simulink model "feedBackCtlPractice1"  (R2020b)
settings: Solver=ode4  StartTime=0.0  StopTime=10.0  FixedStep=0.001  RelTol=1e-3
settings Model: Creator=yuto  LastModifiedBy=yuto
settings DataIOCC: ReturnWorkspaceOutputs=off

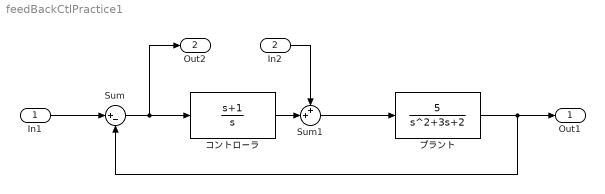
== system feedBackCtlPractice1 ==
  In1 : Inport
  In2 : Inport  Port=2
  Sum : Sum  Inputs=|+-
  Sum1 : Sum  Inputs=++|
  コントローラ : TransferFcn  Numerator=[1 1]  Denominator=[1 0]
  プラント : TransferFcn  Numerator=[5]  Denominator=[1 3 2]
  Out1 : Outport
  Out2 : Outport  Port=2
  wires:
  In1/1 -> Sum/1
  コントローラ/1 -> Sum1/2
  Sum1/1 -> プラント/1
  In2/1 -> Sum1/1
  プラント/1 -> Sum/2, Out1/1
  Sum/1 -> Out2/1, コントローラ/1
